simulink model "Turning_lights"  (R2021a)
settings: Solver=VariableStepAuto  StartTime=0.0  StopTime=10.0  RelTol=1e-3
settings Model: Creator=sampa  LastModifiedBy=sampa

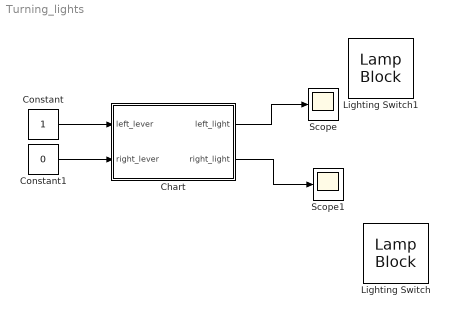
== system Turning_lights ==
  Chart : Stateflow chart  TreatAsAtomicUnit=on
  Constant : Constant
  Constant1 : Constant  Value=0
  Lighting Switch : LampBlock  Icon=LightingSwitch
  Lighting Switch1 : LampBlock  Icon=LightingSwitch
  Scope : Scope
  Scope1 : Scope
  wires:
  Chart/1(left_light) -> Scope/1
  Chart/2(right_light) -> Scope1/1
  Constant/1 -> Chart/1(left_lever)
  Constant1/1 -> Chart/2(right_lever)

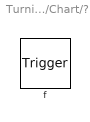
== system Turning_lights/Chart/? ==
  f : TriggerPort  TriggerType=function-call  VariantControl=(inherit)
      settings: CopyFcn=Stateflow.SLINSF.SimulinkMan.removeBlockPreDeleteFcn  PreDeleteFcn=Stateflow.SLINSF.SimulinkMan.unsafePredeleteFcn

== stateflow chart Turning_lights/Chart ==
  state OFF
    entry:
    right_light=0;
    left_light=0;
  state ? [function]
  state LEFT
    state ON
      entry:
      left_light=1;
    state OFF
      entry:
      left_light=0;
    (default) -> LEFT.ON
    LEFT.OFF -> LEFT.ON : after(0.5,sec)
    LEFT.ON -> LEFT.OFF : after(0.5,sec)
  state RIGHT
    state ON
      entry:
      right_light=1;
    state OFF
      entry:
      right_light=0;
    (default) -> RIGHT.ON
    RIGHT.OFF -> RIGHT.ON : after(0.5,sec)
    RIGHT.ON -> RIGHT.OFF : after(0.5,sec)
  (default) -> OFF
  OFF -> LEFT [order 2] : [right_lever==0&&left_lever==1]
  OFF -> RIGHT [order 1] : [right_lever==1&&left_lever==0]
  LEFT -> OFF : [right_lever==0&&left_lever==0]
  RIGHT -> OFF : [right_lever==0&&left_lever==0]
  data: left_lever input; right_lever input; left_light output; right_light output
